simulink model "TrackerMultiObject"  (Simulink 8.4)
settings: Solver=FixedStepDiscrete  StartTime=0.0  StopTime=inf  RelTol=1e-3
libraries: instrumentlib x1
settings Model: Creator=Ssubrama  LastModifiedBy=kpetersen
settings OptimizationCC: InitFltsAndDblsToZero=on
settings GRTTargetCC: TargetFcnLib=ansi_tfl_tmw_new.mat

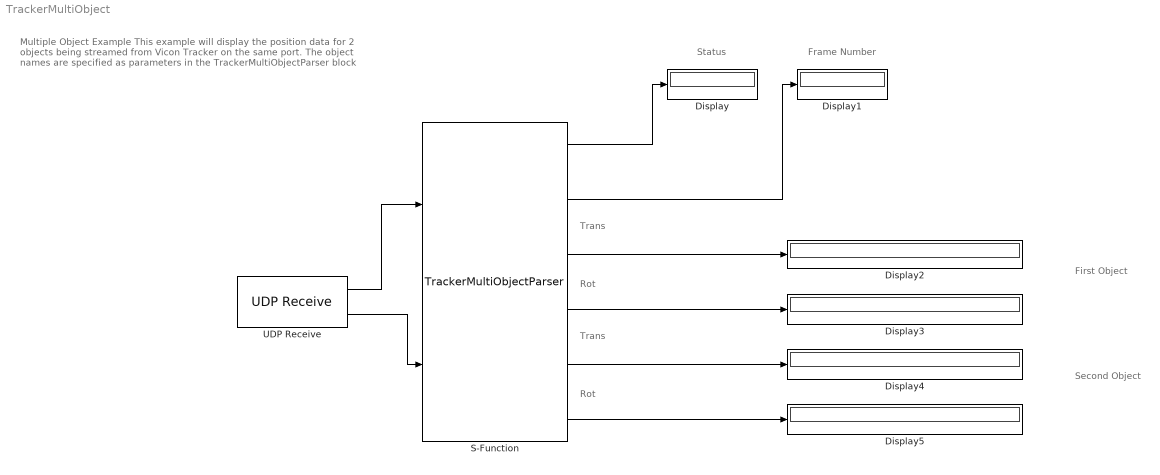
== system TrackerMultiObject ==
  note: Multiple Object Example
      |
      | This example will display the position data
      | for 2 objects being streamed from Vicon
      | Tracker on the same port.
      |
      | The object names are specified as parameters
      | in the TrackerMultiObjectParser block
  note: Frame Number
  note: Status
  note: First Object
  note: Second Object
  note: Trans
  note: Trans
  note: Rot
  note: Rot
  Display{,1..5} (6 alike) : Display
      Display settings: Format=hex (Stored Integer)
  S-Function : S-Function  FunctionName=TrackerMultiObjectParser  Parameters='Object1','Object2'  SFunctionModules=TrackerMultiObjectParser  EnableBusSupport=off
      settings: AttributesFormatString=Data Parser
  UDP Receive : instrumentlib/UDP Receive  Priority=3  Host=localhost  Port=51001  LocalPort=51001  DataSize=256  EnableBlockingMode=off  Timeout=inf  SampleTime=0.01  DataType=uint8  ByteOrder=BigEndian
  wires:
  UDP Receive/1 -> S-Function/1
  S-Function/1 -> Display/1
  UDP Receive/2 -> S-Function/2
  S-Function/2 -> Display1/1
  S-Function/3 -> Display2/1
  S-Function/4 -> Display3/1
  S-Function/5 -> Display4/1
  S-Function/6 -> Display5/1
